simulink model "PID_GM_MessStoer"  (R2021a)
settings: Solver=ode45  StartTime=0.0  StopTime=0.200  RelTol=1e-3  EnableMultiTasking=on
libraries: Regler x2
settings Model: Creator=wll  LastModifiedBy=wll
settings SolverCC: AlgebraicLoopSolver=TrustRegion
settings DataIOCC: LimitDataPoints=on  SaveFormat=Array  SignalLoggingSaveFormat=ModelDataLogs  ReturnWorkspaceOutputs=off
settings OptimizationCC: InitFltsAndDblsToZero=on  LifeSpan=inf
settings DebuggingCC: SaveWithParameterizedLinksMsg=none  UnderspecifiedInitializationDetection=Classic  MergeDetectMultiDrivingBlocksExec=none  SignalResolutionControl=TryResolveAllWithWarning  MultiTaskDSMMsg=warning  MultiTaskCondExecSysMsg=none  SFUnexpectedBacktrackingDiag=warning  SFNoUnconditionalDefaultTransitionDiag=warning  SFExecutionAtInitializationDiag=none  SFMachineParentedDataDiag=warning  ArithmeticOperatorsInVariantConditions=warning
settings HardwareCC: ProdBitPerPointer=32  ProdBitPerSizeT=32  ProdBitPerPtrDiffT=32  ProdLargestAtomicFloat=None  ProdIntDivRoundTo=Undefined  ProdEndianess=Unspecified  ProdWordSize=32  ProdHWDeviceType=32-bit Generic  TargetUnknown=on
settings ModelReferenceCC: PropagateSignalLabelsOutOfModel=off
settings SFSimCC: CustomCodeUndefinedFunction=UseInterfaceOnly
settings CodeAppCC: StateflowObjectComments=on
settings GRTTargetCC: TargetFcnLib=ansi_tfl_tmw.mat  TargetLangStandard=C89/C90 (ANSI)  CombineOutputUpdateFcns=off  GRTInterface=on
settings ConfigComp: CovMetricSettings=dw  CovSaveCumulativeToWorkspaceVar=on  CovSaveSingleToWorkspaceVar=on

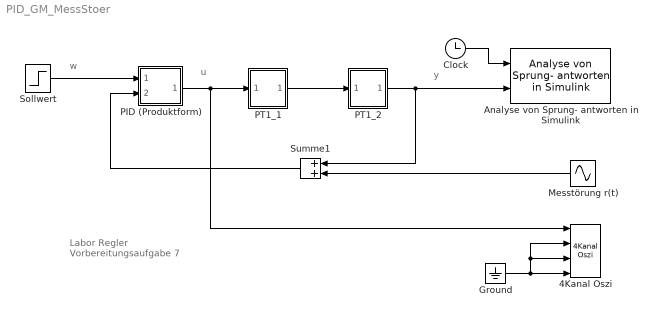
== system PID_GM_MessStoer ==
  note: Labor Regler
      | Vorbereitungsaufgabe 7
  note: w
  note: y
  note: u
  4Kanal Oszi : Regler/4Kanal Oszi  N=20000  k=[1 1 1 1]  y=[-5 5]  tmax=1
  Analyse von Sprung- antworten in Simulink : Regler/Analyse von Sprung- antworten in Simulink  tol=5
  Clock : Clock
  Ground : Ground
  Messtörung r(t) : Sin  Amplitude=0  Frequency=2*pi*2000  SampleTime=0
  PID (Produktform) : Subsystem  mask(PID-Regler in Produktform){kr=2, Ti=0.100, Td=0.005, T1=0}
      mask help: PID(T1) in Produktform kr (1+sTi) (1+sTd) / sTi (1+sT1)
      mask Help:
      | PID-Regler in Produktform mit Proportionalfaktor kr, Integrationszeitkonstante Ti und Differentiationszeitkonstante Td.
      | Der D-Anteil wird durch ein DT1-Glied mit der zusätzlichen Tiefpasszeitkonstante T1 angenähert, es muss sein T1 >= Td/100.
      mask Display: disp('+        \n- PID2')
  PT1_1 : Subsystem  mask(PT1){k=4, T1=0.010}
      mask prompts: k "Verstärkung kp"; T1 "Zeitkonstante T1"
      mask help: PT1-Glied kp/(1+s·T1)
      mask Help: PT1 Tiefpaß 1.Ordnung mit Verstärkung kp und Zeitkonstante T1
      mask Display: disp('PT1')
  PT1_2 : Subsystem  mask(PT1){k=1, T1=0.100}
      mask prompts: k "Verstärkung kp"; T1 "Zeitkonstante T1"
      mask help: PT1-Glied kp/(1+s·T1)
      mask Help: PT1 Tiefpaß 1.Ordnung mit Verstärkung kp und Zeitkonstante T1
      mask Display: disp('PT1')
  Sollwert : Step  Time=0.0001  SampleTime=0
  Summe1 : Sum  InputSameDT=on  SaturateOnIntegerOverflow=on  OutDataTypeStr=Inherit: Same as first input
  wires:
  PT1_2/1(Out1) -> Analyse von Sprung- antworten in Simulink/2, Summe1/1
  PID (Produktform)/1(Stellgröße) -> 4Kanal Oszi/1, PT1_1/1(In1)
  PT1_1/1(Out1) -> PT1_2/1(In1)
  Summe1/1 -> PID (Produktform)/2(Regel- differenz)
  Messtörung r(t)/1 -> Summe1/2
  Sollwert/1 -> PID (Produktform)/1(Regel- differenz1)
  Ground/1 -> 4Kanal Oszi/4, 4Kanal Oszi/2, 4Kanal Oszi/3
  Clock/1 -> Analyse von Sprung- antworten in Simulink/1

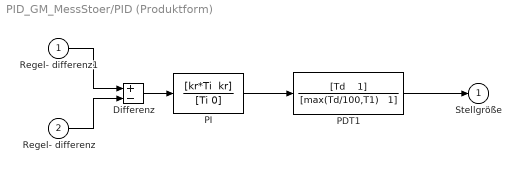
== system PID_GM_MessStoer/PID (Produktform) ==
  Regel- differenz1 : Inport
  Regel- differenz : Inport  Port=2
  Differenz : Sum  Inputs=+-  InputSameDT=on  SaturateOnIntegerOverflow=on  OutDataTypeStr=Inherit: Same as first input
  PDT1 : TransferFcn  Numerator="[Td    1]"  Denominator="[max(Td/100,T1)   1]"
  PI : TransferFcn  Numerator="[kr*Ti  kr]"  Denominator=[Ti 0]
  Stellgröße : Outport  VectorParamsAs1DForOutWhenUnconnected=off
  wires:
  Regel- differenz1/1 -> Differenz/1
  Regel- differenz/1 -> Differenz/2
  Differenz/1 -> PI/1
  PI/1 -> PDT1/1
  PDT1/1 -> Stellgröße/1

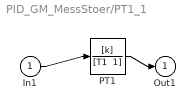
== system PID_GM_MessStoer/PT1_1 ==
  In1 : Inport
  PT1 : TransferFcn  Numerator=[k]  Denominator="[T1  1]"
  Out1 : Outport  VectorParamsAs1DForOutWhenUnconnected=off
  wires:
  In1/1 -> PT1/1
  PT1/1 -> Out1/1

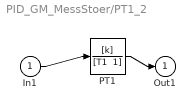
== system PID_GM_MessStoer/PT1_2 ==
  In1 : Inport
  PT1 : TransferFcn  Numerator=[k]  Denominator="[T1  1]"
  Out1 : Outport  VectorParamsAs1DForOutWhenUnconnected=off
  wires:
  PT1/1 -> Out1/1
  In1/1 -> PT1/1
